simulink model "assignment4"  (R2017a)
settings: Solver=VariableStepAuto  StartTime=0.0  StopTime=10  RelTol=1e-3
undefined symbols (not defined in the file): sigbuilder_block
libraries: fl_lib x26, nesl_utility x24, pe_lib x11, elec_lib x6, powerlib_meascontrol x3
settings Model: Creator=hxx733  LastModifiedBy=super

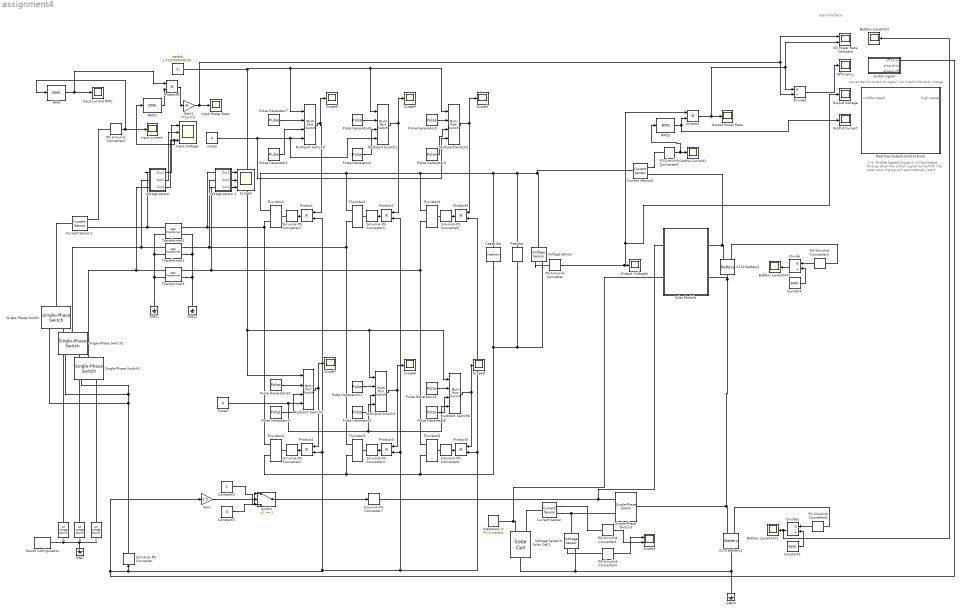
== system assignment4 ==
  note: User Interface
  note: remember to switch to signal 1 to check the solar charge
  note: high speed
  note: middle speed
  note: 1~2: Middle Speed Charge
      | 2~3:Fast Speed Charge
      | when the switch signal turned off,
      | the solar slow charge will automatically start.
  " Output Power Rate" : Scope
  " product " : Product
  2170 Battery1 : elec_lib/Sources/Battery  Vnom=3.7 V  R1=0.05 Ohm  prm_AH=2  AH=5.75 hr*A  V1=3 V  AH1=1.15 hr*A  prm_R2=1  R2=2000 Ohm  prm_fade=1  N_fade=100  AH_fade=45 hr*A  R1_fade=2.02 Ohm  V1_fade=10.35 V  i_specify=off  i_priority=None  i=0 A  i_nominal_specify=off  i_nominal_unit=A  i_nominal_value=1  v_specify=off  v_priority=None  v=0 V  v_nominal_specify=off  v_nominal_unit=V  v_nominal_value=1  charge_specify=on  charge_priority=High  charge=0 hr*A  charge_nominal_specify=off  charge_nominal_unit=hr*A  charge_nominal_value=1  num_cycles_specify=off  num_cycles_priority=High  num_cycles=0  num_cycles_nominal_specify=off  num_cycles_nominal_unit=1  num_cycles_nominal_value=1  thermal_mass=30000 J/K  Tmeas=298.15 K  Vnom_T2=12 V  R1_T2=2.2 Ohm  V1_T2=11.4 V  R2_T2=2200 Ohm  Tmeas2=273.15 K  temperature_specify=off  temperature_priority=High  temperature=298.15 K  temperature_nominal_specify=off  temperature_nominal_unit=K  temperature_nominal_value=1
      settings: SourceProductName=Simscape Electronics  SourceProductBaseCode=SN
  2170 Battery2 : elec_lib/Sources/Battery  Vnom=3.7 V  R1=0.05 Ohm  prm_AH=2  AH=5.75 hr*A  V1=3 V  AH1=1.15 hr*A  prm_R2=1  R2=2000 Ohm  prm_fade=1  N_fade=100  AH_fade=45 hr*A  R1_fade=2.02 Ohm  V1_fade=10.35 V  i_specify=off  i_priority=None  i=0 A  i_nominal_specify=off  i_nominal_unit=A  i_nominal_value=1  v_specify=off  v_priority=None  v=0 V  v_nominal_specify=off  v_nominal_unit=V  v_nominal_value=1  charge_specify=on  charge_priority=High  charge=0 hr*A  charge_nominal_specify=off  charge_nominal_unit=hr*A  charge_nominal_value=1  num_cycles_specify=off  num_cycles_priority=High  num_cycles=0  num_cycles_nominal_specify=off  num_cycles_nominal_unit=1  num_cycles_nominal_value=1  thermal_mass=30000 J/K  Tmeas=298.15 K  Vnom_T2=12 V  R1_T2=2.2 Ohm  V1_T2=11.4 V  R2_T2=2200 Ohm  Tmeas2=273.15 K  temperature_specify=off  temperature_priority=High  temperature=298.15 K  temperature_nominal_specify=off  temperature_nominal_unit=K  temperature_nominal_value=1
      settings: SourceProductName=Simscape Electronics  SourceProductBaseCode=SN
  A : fl_lib/Electrical/Electrical Sources/AC Voltage Source  amp=380/sqrt(3) V  shift=0 deg  frequency=50 Hz  omega=0 rad/s
  B : fl_lib/Electrical/Electrical Sources/AC Voltage Source  amp=380/sqrt(3) V  shift=120 deg  frequency=50 Hz  omega=0 rad/s
  Battery Level(Ah) : Scope
  Battery Level(Ah)1 : Scope
  Battery Level3(Ah) : Scope
  C : fl_lib/Electrical/Electrical Sources/AC Voltage Source  amp=380/sqrt(3) V  shift=240 deg  frequency=50 Hz  omega=0 rad/s
  Capacitor : elec_lib/Passive Devices/Capacitor  enable_table=0  c=100e-6 F  Cvec=[1.0e-5, 1.0e-6] F  Vvec=[0.0, 10.0] V  CV_table_symmetry=1  C_tol=5  enable_C_tol=0  tol_distribution=1  nSigma=4  r=1e-6 Ohm  g=0 1/Ohm  enable_operating_limits=0  operating_limit_action=2  max_working_voltage_range=[-25.0, 25.0] V  power_rating=1 W  enable_faults=0  fault_action=1  Cscale_faulted=100  R_faulted=1e-3 Ohm  G_faulted=0 1/Ohm  tau_fault=1e-3 s  enable_temporal_fault=0  t_fault=1 s  enable_behavioral_fault=0  max_permissible_voltage_range=[-100.0, 100.0] V  t_fail_on_voltage=1 s  i_specify=off  i_priority=None  i=0 A  i_nominal_specify=off  i_nominal_unit=A  i_nominal_value=1  v_specify=off  v_priority=None  v=0 V  v_nominal_specify=off  v_nominal_unit=V  v_nominal_value=1  vc_specify=off  vc_priority=High  vc=0 V  vc_nominal_specify=off  vc_nominal_unit=V  vc_nominal_value=1
  Constant : Constant  Value=3600
  Constant1 : Constant  Value=3600
  Constant2 : Constant
  Constant3 : Constant  Value=0
  Current Sensor : fl_lib/Electrical/Electrical Sensors/Current Sensor
  Current Sensor1 : fl_lib/Electrical/Electrical Sensors/Current Sensor
  Current Sensor2 : fl_lib/Electrical/Electrical Sensors/Current Sensor
  Divide : Product  Inputs=*/
  Divide1 : Product  Inputs=*/
  Divide2 : Product  Inputs=*/
  Efficiency : Scope
  GND{,1..2,4} (4 alike) : fl_lib/Electrical/Electrical Elements/Electrical Reference
  Gain : Gain  Gain=1.5
  Gain1 : Gain  Gain=3*sqrt(3)
  I/O Power Rate Compare : Scope  NumInputPorts=2
  Input Power Rate : Scope
  Input Voltage : Scope  NumInputPorts=3
  Input current : Scope
  Input current RMS : Scope
  "Irradiance, Ir" : fl_lib/Physical Signals/Sources/PS Constant  constant=1900*10
      settings: SourceProductName=Foundation Library
  Multiport Switch{1..6} (6 alike) : MultiPortSwitch
  OutPut Current : Scope
  OutPut Current1 : Scope
  Output Voltage : Scope
  Output Voltage1 : Scope
  PS-Simulink Converter{,1,3..4,6} (5 alike) : nesl_utility/PS-Simulink Converter  PhysicalDomain=network_engine_domain  SubClassName=ps_output  LeftPortType=input  RightPortType=output  PseudoPeriodic=off  Frequencies=[]  Unit=1  AffineConversion=off
  PS-Simulink Converter2 : nesl_utility/PS-Simulink Converter  PhysicalDomain=network_engine_domain  SubClassName=ps_output  LeftPortType=input  RightPortType=output  PseudoPeriodic=off  Frequencies=[]  Unit=C  AffineConversion=off
  PS-Simulink Converter5 : nesl_utility/PS-Simulink Converter  PhysicalDomain=network_engine_domain  SubClassName=ps_output  LeftPortType=input  RightPortType=output  PseudoPeriodic=off  Frequencies=[]  Unit=C  AffineConversion=off
  Product{,1..6} (7 alike) : Product
  Pulse Generator1 : DiscretePulseGenerator  PulseType=Time based  Period=1/50  PulseWidth=50
  Pulse Generator10 : DiscretePulseGenerator  PulseType=Time based  Period=1/50  PulseWidth=50  PhaseDelay=3/50/6++1/50/4
  Pulse Generator11 : DiscretePulseGenerator  PulseType=Time based  Period=1/50  PulseWidth=50  PhaseDelay=1/50/6+1/50/4
  Pulse Generator12 : DiscretePulseGenerator  PulseType=Time based  Period=1/50  PulseWidth=50  PhaseDelay=5/50/6+1/50/4
  Pulse Generator2 : DiscretePulseGenerator  PulseType=Time based  Period=1/50  PulseWidth=50  PhaseDelay=4/50/6
  Pulse Generator3 : DiscretePulseGenerator  PulseType=Time based  Period=1/50  PulseWidth=50  PhaseDelay=2/50/6
  Pulse Generator4 : DiscretePulseGenerator  PulseType=Time based  Period=1/50  PulseWidth=50  PhaseDelay=3/50/6
  Pulse Generator5 : DiscretePulseGenerator  PulseType=Time based  Period=1/50  PulseWidth=50  PhaseDelay=1/50/6
  Pulse Generator6 : DiscretePulseGenerator  PulseType=Time based  Period=1/50  PulseWidth=50  PhaseDelay=5/50/6
  Pulse Generator7 : DiscretePulseGenerator  PulseType=Time based  Period=1/50  PulseWidth=50  PhaseDelay=0+1/50/4
  Pulse Generator8 : DiscretePulseGenerator  PulseType=Time based  Period=1/50  PulseWidth=50  PhaseDelay=4/50/6+1/50/4
  Pulse Generator9 : DiscretePulseGenerator  PulseType=Time based  Period=1/50  PulseWidth=50  PhaseDelay=2/50/6+1/50/4
  RMS : powerlib_meascontrol/Measurements/RMS  TrueRMS=on  Freq=50  RMSInit=120  Ts=0
  RMS1 : powerlib_meascontrol/Measurements/RMS  TrueRMS=on  Freq=50  RMSInit=120  Ts=0
  RMS2 : powerlib_meascontrol/Measurements/RMS  TrueRMS=on  Freq=50  RMSInit=120  Ts=0
  Rectifier Output Control Knob : Subsystem  DialogController=hmiCreateDDGDialog  IsWebBlock=on  mask(MWDashboardBlock){webBlockId=5efd5572-5288-454e-8a17-a3fe679787e4, webBlockType=continuousknob, ShowInLibBrowser=on, ShowInitialText=on, HMISrcModelName=individualfinished}
      mask prompts: webBlockId "WebBlock Id"; webBlockType "WebBlock Type"; HMISrcModelName "Source Model"
      mask Help: helpview([docroot '/mapfiles/simulink.map'], 'hmi_knob')
      mask Display:
      | if strcmp(get_param(bdroot(gcb),'BlockDiagramType'), 'library')
      |     image([(matlabroot) '/toolbox/simulink/hmi/icons/ContinuousKnob.png']);
      | end
  Resistor : elec_lib/Passive Devices/Resistor  R=100 kOhm  R_tol=5  enable_R_tol=0  tol_distribution=1  nSigma=4  enable_operating_limits=0  operating_limit_action=2  max_working_voltage=100 V  power_rating=1 W  enable_faults=0  fault_action=1  R_faulted=inf Ohm  enable_temporal_fault=0  t_fault=1 s  enable_behavioral_fault=0  max_permissible_current=1 A  t_fail_on_current=1 s  noise_mode=0  sample_time=1e-3 s  repeatability=1  auto_seed=2769242599  user_seed=0  Tdevice=25 degC  alpha=3.93e-3 1/K  Tmeas=25 degC  thermal_mass=100 J/K  power_derating_T1=70 degC  power_derating_T2=155 degC  operating_temperature_range_vec=[-50.0, 150.0] degC  temperature_specify=off  temperature_priority=High  temperature=298.15 K  temperature_nominal_specify=off  temperature_nominal_unit=K  temperature_nominal_value=1
  Scope2 : Scope  NumInputPorts=3
  Scope3 : Scope  NumInputPorts=2
  Scope{4..9} (6 alike) : Scope
  Simulink-PS Converter{,1..7} (8 alike) : nesl_utility/Simulink-PS Converter  PhysicalDomain=network_engine_domain  SubClassName=ps_input  LeftPortType=input  RightPortType=output  PseudoPeriodic=off  Frequencies=[]  NoiseDistribution=none  NoiseParameters=[]  Unit=1  AffineConversion=off  FilteringAndDerivatives=provide  SimscapeFilterOrder=1  InputFilterTimeConstant=0.001  UdotUserProvided=0
  Single-Phase Switch{,1..3} (4 alike) : pe_lib/Switches & Breakers/Fundamental Components/Single-Phase Switch  R_closed=0.001 Ohm  G_open=1e-6 1/Ohm  threshold=0 V
      settings: SourceProductName=Simscape Power Systems  SourceProductBaseCode=PS
  Solar Cell1 : elec_lib/Sources/Solar Cell  prm=3  Isc=3.8 A  Voc=0.586 V  Is=3.15e-07 A  Is2=0 A  Iph=3.80 A  Ir0=1000 W/m^2  ec=1.4  N2=2  Rs=0.0042 Ohm  Rp=10.1 Ohm  N_series=700  TIPH1=0.000805 1/K  EG=1.14 eV  TXIS1=3.38  TXIS2=3  TRS1=0  TRP1=0  Tmeas=25 degC  TFIXED=30 degC  thermal_mass=100 J/K  initial_temperature=25 degC
      settings: SourceProductName=Simscape Electronics  SourceProductBaseCode=SN
  Solar Module : Subsystem
  Solver Configuration : nesl_utility/Solver Configuration  PhysicalDomain=network_engine_domain  SubClassName=solver  LeftPortType=input  RightPortType=generic  Accelerate=off  Tones=[]  Harmonics=[]  SimulateNoise=off  Profile=off  UseLocalSampling=off  EnableSwitchedLinearOptims=on  FrequencyDomain=off  UseCCode=off  RelTol=0.001  AbsTol=1e-06  MinStep=1e-09  ToWorkspace=off  RevertToSquareIcSolve=off  NumHomotopyIterations=100  PhasorMode=off  PhasorModeNumHarmonics=1  OverrideAbsTol=off  DoDC=off  ResidualTolerance=1e-09  UseLocalSolver=off  LocalSolverChoice=NE_BACKWARD_EULER_ADVANCER  LocalSolverSampleTime=0.001  DoFixedCost=off  MaxNonlinIter=3  MaxModeIter=2  LinearAlgebra=Sparse  DelaysMemoryBudget=1024  AutomaticFiltering=on  FilteringTimeConstant=0.001
  Switch : Switch  Threshold=1
  Thyristor{1..6} (6 alike) : pe_lib/Semiconductors/Fundamental Components/Thyristor  Vf=0.8 V  Ron=0.001 Ohm  Goff=1e-5 1/Ohm  Vgt=0.5 V  Ih=1 A  diode_param=1  diode_Vf=0.8 V  diode_Ron=0.001 Ohm  diode_Goff=1e-5 1/Ohm  diode_C=5e-8 F  diode_iRM=-235 A  diode_iF=300 A  diode_idot=-50 A/us  diode_trr_param=1  diode_trr_factor=3  diode_trr=15 us  diode_Qrr=1.5e+3 s*uA  thermal_loss_option=2  Voff=300 V  Tau=1e-4 s  Tj=[ 298.15 398.15 ] K  Iout_scalar=600 A  Eon_scalar=0.02286 J  Eoff_scalar=0.01714 J  Von_scalar=2.7 V  Iout_data=[ 0 10 50 100 200 400 600 ] A  Eon_data=[ 0 2.9e-4 0.00143 0.00286 0.00571 0.01314 0.02286; 0 5.7e-4 0.00263 0.00514 0.01029 0.02057 0.03029 ] J  Eoff_data=[ 0 2.1e-4 0.00107 0.00214 0.00429 0.009859999999999999 0.01714; 0 4.3e-4 0.00197 0.00386 0.00771 0.01543 0.02271 ] J  Von_data=[ 0 1.1 1.3 1.45 1.75 2.25 2.7; 0 1 1.15 1.35 1.7 2.35 3 ] V
      settings: SourceProductName=Simscape Power Systems  SourceProductBaseCode=PS
  Transformer1 : fl_lib/Electrical/Electrical Elements/Ideal Transformer  n=1:1  i1_specify=off  i1_priority=None  i1=0 A  i1_nominal_specify=off  i1_nominal_unit=A  i1_nominal_value=1  v1_specify=off  v1_priority=None  v1=0 V  v1_nominal_specify=off  v1_nominal_unit=V  v1_nominal_value=1  i2_specify=off  i2_priority=None  i2=0 A  i2_nominal_specify=off  i2_nominal_unit=A  i2_nominal_value=1  v2_specify=off  v2_priority=None  v2=0 V  v2_nominal_specify=off  v2_nominal_unit=V  v2_nominal_value=1
      settings: SourceProductName=Simscape  SourceProductBaseCode=SS
  Transformer2 : fl_lib/Electrical/Electrical Elements/Ideal Transformer  n=1:1  i1_specify=off  i1_priority=None  i1=0 A  i1_nominal_specify=off  i1_nominal_unit=A  i1_nominal_value=1  v1_specify=off  v1_priority=None  v1=0 V  v1_nominal_specify=off  v1_nominal_unit=V  v1_nominal_value=1  i2_specify=off  i2_priority=None  i2=0 A  i2_nominal_specify=off  i2_nominal_unit=A  i2_nominal_value=1  v2_specify=off  v2_priority=None  v2=0 V  v2_nominal_specify=off  v2_nominal_unit=V  v2_nominal_value=1
      settings: SourceProductName=Simscape  SourceProductBaseCode=SS
  Transformer3 : fl_lib/Electrical/Electrical Elements/Ideal Transformer  n=1:1  i1_specify=off  i1_priority=None  i1=0 A  i1_nominal_specify=off  i1_nominal_unit=A  i1_nominal_value=1  v1_specify=off  v1_priority=None  v1=0 V  v1_nominal_specify=off  v1_nominal_unit=V  v1_nominal_value=1  i2_specify=off  i2_priority=None  i2=0 A  i2_nominal_specify=off  i2_nominal_unit=A  i2_nominal_value=1  v2_specify=off  v2_priority=None  v2=0 V  v2_nominal_specify=off  v2_nominal_unit=V  v2_nominal_value=1
      settings: SourceProductName=Simscape  SourceProductBaseCode=SS
  Voltage Sensor : fl_lib/Electrical/Electrical Sensors/Voltage Sensor
  Voltage Sensor4 : fl_lib/Electrical/Electrical Sensors/Voltage Sensor
  none1 : Constant  Value=0
  none2 : Constant  Value=0
  switch : Constant  Value=2.4320085608106
  switch signal : Subsystem  Tag=STV Subsys  LoadFcn=sigbuilder_block('load');  StartFcn=sigbuilder_block('start');  StopFcn=sigbuilder_block('stop');  ClipboardFcn=sigbuilder_block('clipboard');  mask(Sigbuilder block){tuvar=[0:10]}
      mask help: Simulink:masks:SigbuilderBlock_MD
      mask init:
      | if ~strcmp(get_param(bdroot(gcbh),'SimulationStatus'),'stopped') tuvar = sigbuilder_block('maskInit'); end
      settings: CopyFcn=sigbuilder_block('copy');  DeleteFcn=sigbuilder_block('delete');  ModelCloseFcn=sigbuilder_block('modelClose');  PreSaveFcn=sigbuilder_block('preSave');  PauseFcn=sigbuilder_block('pause');  ContinueFcn=sigbuilder_block('continue');  NameChangeFcn=sigbuilder_block('namechange');  OpenFcn=sigbuilder_block('open',[442.125 105 550.5 400.125 ]);  CloseFcn=sigbuilder_block('close');
      mask Display: plot(0, 0, 100, 100,[2, 2, 32, 32, 2], [68, 8, 8, 68, 68],[32, 2], [38, 38], [32, 19, 2],[53, 60, 44], [32, 17, 17, 2],[16, 16, 31, 31]);txt = getActiveGroup(gcbh);text(2, 100, txt,'verticalAlignment', 'top');
  "voltage sensor " : Subsystem
  voltage sensor 1 : Subsystem
  wires:
  PS-Simulink Converter/1 -> Output Voltage/1, " product "/1, Output Voltage1/1
  PS-Simulink Converter4/1 -> Scope3/1
  "voltage sensor "/1(Out1) -> Input Voltage/1
  "voltage sensor "/2(Out2) -> Input Voltage/2
  "voltage sensor "/3(Out3) -> RMS1/1, Input Voltage/3
  PS-Simulink Converter1/1 -> Scope3/2
  Product/1 -> Simulink-PS Converter1/1
  Product1/1 -> Simulink-PS Converter2/1
  Product2/1 -> Simulink-PS Converter3/1
  Product3/1 -> Simulink-PS Converter4/1
  Product4/1 -> Simulink-PS Converter5/1
  Product5/1 -> Simulink-PS Converter6/1
  Divide/1 -> Battery Level3(Ah)/1
  PS-Simulink Converter5/1 -> Divide/1
  Constant/1 -> Divide/2
  PS-Simulink Converter2/1 -> Divide1/1
  Constant1/1 -> Divide1/2
  Divide1/1 -> Battery Level(Ah)/1, Battery Level(Ah)1/1
  Multiport Switch1/1 -> Product2/1, Scope4/1
  Pulse Generator2/1 -> Multiport Switch1/3
  Pulse Generator8/1 -> Multiport Switch1/2
  Pulse Generator3/1 -> Multiport Switch2/3
  Pulse Generator9/1 -> Multiport Switch2/2
  Multiport Switch2/1 -> Product4/1, Scope5/1
  none1/1 -> Multiport Switch2/4, Multiport Switch1/4, Multiport Switch3/4
  Multiport Switch3/1 -> Product/1, Scope6/1
  Pulse Generator1/1 -> Multiport Switch3/3
  Pulse Generator7/1 -> Multiport Switch3/2
  Multiport Switch4/1 -> Product1/1, Scope7/1
  none2/1 -> Multiport Switch4/4, Multiport Switch6/4, Multiport Switch5/4
  Pulse Generator10/1 -> Multiport Switch4/2
  Pulse Generator4/1 -> Multiport Switch4/3
  Multiport Switch5/1 -> Product3/1, Scope8/1
  Pulse Generator11/1 -> Multiport Switch5/2
  Pulse Generator5/1 -> Multiport Switch5/3
  Multiport Switch6/1 -> Product5/1, Scope9/1
  Pulse Generator12/1 -> Multiport Switch6/2
  Pulse Generator6/1 -> Multiport Switch6/3
  voltage sensor 1/1(Out1) -> Scope2/1
  voltage sensor 1/3(Out3) -> Scope2/3
  voltage sensor 1/2(Out2) -> Scope2/2
  Constant3/1 -> Switch/1
  Constant2/1 -> Switch/3
  Gain/1 -> Switch/2
  switch signal/1(off to on) -> Gain/1, Product/2, Product1/2, Product2/2, Product3/2, Product4/2, Product5/2, Simulink-PS Converter/1
  switch/1 -> Multiport Switch4/1, Multiport Switch6/1, Multiport Switch5/1, Multiport Switch3/1, Multiport Switch2/1, Multiport Switch1/1
  Switch/1 -> Simulink-PS Converter7/1
  PS-Simulink Converter3/1 -> RMS/1, Input current/1
  Product6/1 -> Gain1/1
  Gain1/1 -> Divide2/2, I/O Power Rate Compare/1, Input Power Rate/1
  PS-Simulink Converter6/1 -> RMS2/1, OutPut Current1/1
  " product "/1 -> Divide2/1, I/O Power Rate Compare/2, " Output Power Rate"/1
  Divide2/1 -> Efficiency/1
  RMS/1 -> Product6/1, Input current RMS/1
  RMS1/1 -> Product6/2
  RMS2/1 -> " product "/2, OutPut Current/1
  connections:
  B/RConn1 -- Solver Configuration/RConn1 -- A/RConn1 -- C/RConn1 -- GND/LConn1
  GND1/LConn1 -- Transformer3/LConn2 -- Transformer1/LConn2 -- Transformer2/LConn2
  Transformer2/RConn2 -- Transformer1/RConn2 -- Transformer3/RConn2 -- GND2/LConn1
  "voltage sensor "/LConn2 -- Single-Phase Switch1/RConn1 -- Transformer2/LConn1
  "voltage sensor "/LConn1 -- Transformer1/LConn1 -- Current Sensor1/RConn2
  Thyristor1/RConn1 -- voltage sensor 1/LConn1 -- Transformer1/RConn1 -- Thyristor4/RConn2
  Thyristor2/RConn1 -- voltage sensor 1/LConn2 -- Transformer2/RConn1 -- Thyristor5/RConn2
  Thyristor3/RConn1 -- Transformer3/RConn1 -- voltage sensor 1/LConn3 -- Thyristor6/RConn2
  Thyristor4/RConn1 -- Thyristor5/RConn1 -- Voltage Sensor/RConn2 -- Resistor/RConn1 -- Capacitor/RConn1 -- Thyristor6/RConn1
  Voltage Sensor/RConn1 -- PS-Simulink Converter/LConn1
  Solar Module/LConn2 -- Solar Cell1/LConn1 -- "Irradiance, Ir"/RConn1
  Voltage Sensor4/RConn1 -- PS-Simulink Converter4/LConn1
  Voltage Sensor/LConn1 -- Current Sensor2/LConn1 -- Resistor/LConn1 -- Thyristor1/RConn2 -- Thyristor2/RConn2 -- Thyristor3/RConn2 -- Capacitor/LConn1
  Voltage Sensor4/RConn2 -- Solar Cell1/RConn1 -- 2170 Battery2/RConn1 -- GND4/LConn1
  2170 Battery2/LConn1 -- Solar Module/RConn2 -- 2170 Battery1/RConn1 -- Single-Phase Switch3/RConn1
  "voltage sensor "/LConn3 -- Single-Phase Switch2/RConn1 -- Transformer3/LConn1
  Current Sensor/LConn1 -- Solar Cell1/LConn2
  Current Sensor/RConn1 -- PS-Simulink Converter1/LConn1
  A/LConn1 -- Single-Phase Switch/LConn2
  B/LConn1 -- Single-Phase Switch1/LConn2
  Single-Phase Switch2/LConn2 -- C/LConn1
  Simulink-PS Converter/RConn1 -- Single-Phase Switch2/LConn1 -- Single-Phase Switch1/LConn1 -- Single-Phase Switch/LConn1
  Simulink-PS Converter1/RConn1 -- Thyristor1/LConn1
  Simulink-PS Converter2/RConn1 -- Thyristor4/LConn1
  Simulink-PS Converter3/RConn1 -- Thyristor2/LConn1
  Simulink-PS Converter4/RConn1 -- Thyristor5/LConn1
  Simulink-PS Converter5/RConn1 -- Thyristor3/LConn1
  Simulink-PS Converter6/RConn1 -- Thyristor6/LConn1
  2170 Battery1/LConn2 -- PS-Simulink Converter5/LConn1
  Current Sensor/RConn2 -- Single-Phase Switch3/LConn2 -- Voltage Sensor4/LConn1
  2170 Battery2/LConn2 -- PS-Simulink Converter2/LConn1
  Simulink-PS Converter7/RConn1 -- Solar Module/LConn1 -- Single-Phase Switch3/LConn1
  Current Sensor1/LConn1 -- Single-Phase Switch/RConn1
  Current Sensor1/RConn1 -- PS-Simulink Converter3/LConn1
  Solar Module/RConn1 -- Current Sensor2/RConn2 -- 2170 Battery1/LConn1
  Current Sensor2/RConn1 -- PS-Simulink Converter6/LConn1

== system assignment4/Rectifier Output Control Knob ==

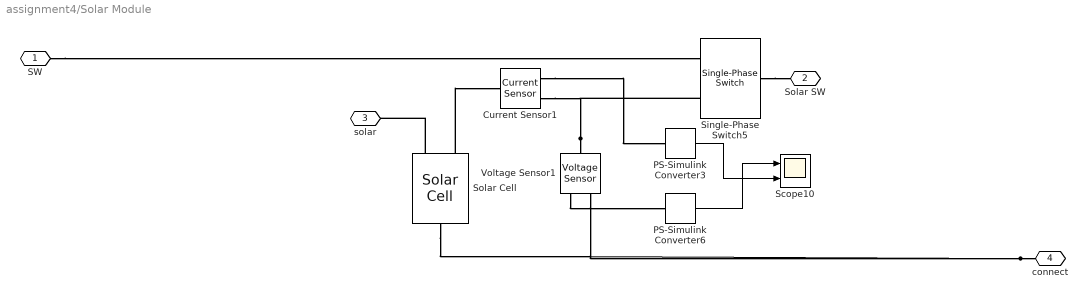
== system assignment4/Solar Module ==
  Current Sensor1 : fl_lib/Electrical/Electrical Sensors/Current Sensor
  PS-Simulink Converter3 : nesl_utility/PS-Simulink Converter  PhysicalDomain=network_engine_domain  SubClassName=ps_output  LeftPortType=input  RightPortType=output  PseudoPeriodic=off  Frequencies=[]  Unit=1  AffineConversion=off
  PS-Simulink Converter6 : nesl_utility/PS-Simulink Converter  PhysicalDomain=network_engine_domain  SubClassName=ps_output  LeftPortType=input  RightPortType=output  PseudoPeriodic=off  Frequencies=[]  Unit=1  AffineConversion=off
  Scope10 : Scope  NumInputPorts=2
  Single-Phase Switch5 : pe_lib/Switches & Breakers/Fundamental Components/Single-Phase Switch  R_closed=0.001 Ohm  G_open=1e-6 1/Ohm  threshold=0 V
      settings: SourceProductName=Simscape Power Systems  SourceProductBaseCode=PS
  Solar Cell : elec_lib/Sources/Solar Cell  prm=3  Isc=3.8 A  Voc=0.586 V  Is=3.15e-07 A  Is2=0 A  Iph=3.80 A  Ir0=1000 W/m^2  ec=1.4  N2=2  Rs=0.0042 Ohm  Rp=10.1 Ohm  N_series=700  TIPH1=0.000805 1/K  EG=1.14 eV  TXIS1=3.38  TXIS2=3  TRS1=0  TRP1=0  Tmeas=25 degC  TFIXED=30 degC  thermal_mass=100 J/K  initial_temperature=25 degC
      settings: SourceProductName=Simscape Electronics  SourceProductBaseCode=SN
  Voltage Sensor1 : fl_lib/Electrical/Electrical Sensors/Voltage Sensor
  SW : PMIOPort  Port=1  Side=Left
  Solar SW : PMIOPort  Port=2  Side=Right
  solar : PMIOPort  Port=3  Side=Left
  connect : PMIOPort  Port=4  Side=Right
  wires:
  PS-Simulink Converter3/1 -> Scope10/2
  PS-Simulink Converter6/1 -> Scope10/1
  connections:
  Voltage Sensor1/RConn1 -- PS-Simulink Converter6/LConn1
  Voltage Sensor1/LConn1 -- Current Sensor1/RConn2 -- Single-Phase Switch5/LConn2
  Solar Cell/LConn2 -- Current Sensor1/LConn1
  SW/RConn1 -- Single-Phase Switch5/LConn1
  Current Sensor1/RConn1 -- PS-Simulink Converter3/LConn1
  connect/RConn1 -- Solar Cell/RConn1 -- Voltage Sensor1/RConn2
  Solar Cell/LConn1 -- solar/RConn1
  Single-Phase Switch5/RConn1 -- Solar SW/RConn1

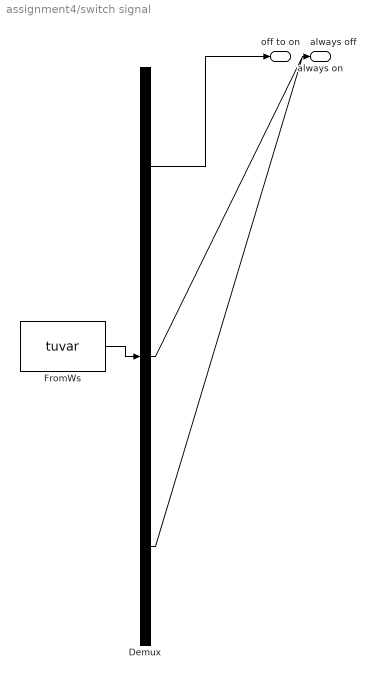
== system assignment4/switch signal ==
  Demux : Demux  Tag=STV Demux  Outputs=3
  FromWs : FromWorkspace  Tag=STV FromWs  VariableName=tuvar  SampleTime=0
      SigBuilderData=|
      | common.afterFinalStr = 'Extrapolate'
      | common.sampleTime = 0
      | dataSet.timeRange = [0 10]
      | dataSet.name = 'Group 1'
      | sbobj.Groups.Name = 'Group 1'
      | sbobj.Groups.Signals(1).Name = 'off to on'
      | sbobj.Groups.Signals(1).XData = [0 5 5 6 10]
      | sbobj.Groups.Signals(1).YData = [0 0 0.995 0.995 0.995]
      | sbobj.Groups.Signals(2).Name = 'always on'
      | sbobj.Groups.Signals(2).XData = [0 10]
      | sbobj.Groups.Signals(2).YData = [1 1]
      | sbobj.Groups.Signals(3).Name = 'always off'
      | sbobj.Groups.Signals(3).XData = [0 10]
      | sbobj.Groups.Signals(3).YData = [0 0]
  off to on : Outport  Tag=STV Outport
  always on : Outport  Tag=STV Outport  Port=2
  always off : Outport  Tag=STV Outport  Port=3
  wires:
  Demux/1 -> off to on/1
  FromWs/1 -> Demux/1
  Demux/2 -> always on/1
  Demux/3 -> always off/1

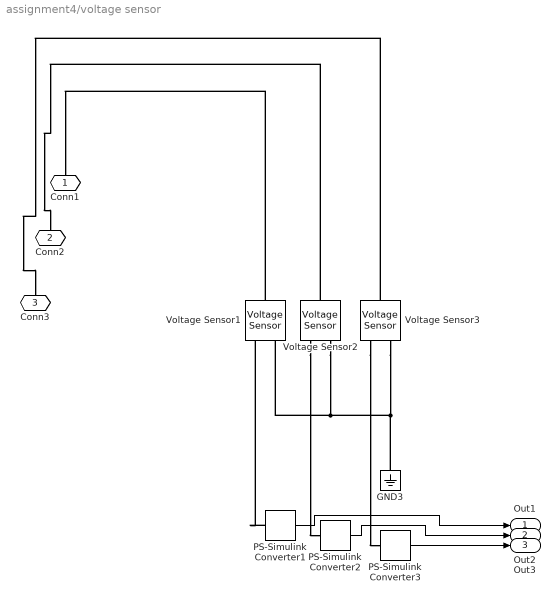
== system assignment4/voltage sensor  ==
  GND3 : fl_lib/Electrical/Electrical Elements/Electrical Reference
  PS-Simulink Converter1 : nesl_utility/PS-Simulink Converter  PhysicalDomain=network_engine_domain  SubClassName=ps_output  LeftPortType=input  RightPortType=output  PseudoPeriodic=off  Frequencies=[]  Unit=1  AffineConversion=off
  PS-Simulink Converter2 : nesl_utility/PS-Simulink Converter  PhysicalDomain=network_engine_domain  SubClassName=ps_output  LeftPortType=input  RightPortType=output  PseudoPeriodic=off  Frequencies=[]  Unit=1  AffineConversion=off
  PS-Simulink Converter3 : nesl_utility/PS-Simulink Converter  PhysicalDomain=network_engine_domain  SubClassName=ps_output  LeftPortType=input  RightPortType=output  PseudoPeriodic=off  Frequencies=[]  Unit=1  AffineConversion=off
  Voltage Sensor1 : fl_lib/Electrical/Electrical Sensors/Voltage Sensor
  Voltage Sensor2 : fl_lib/Electrical/Electrical Sensors/Voltage Sensor
  Voltage Sensor3 : fl_lib/Electrical/Electrical Sensors/Voltage Sensor
  Conn1 : PMIOPort  Port=1  Side=Left
  Conn2 : PMIOPort  Port=2  Side=Left
  Conn3 : PMIOPort  Port=3  Side=Left
  Out1 : Outport
  Out2 : Outport  Port=2
  Out3 : Outport  Port=3
  wires:
  PS-Simulink Converter1/1 -> Out1/1
  PS-Simulink Converter2/1 -> Out2/1
  PS-Simulink Converter3/1 -> Out3/1
  connections:
  Voltage Sensor3/LConn1 -- Conn3/RConn1
  GND3/LConn1 -- Voltage Sensor2/RConn2 -- Voltage Sensor1/RConn2 -- Voltage Sensor3/RConn2
  PS-Simulink Converter1/LConn1 -- Voltage Sensor1/RConn1
  Voltage Sensor2/RConn1 -- PS-Simulink Converter2/LConn1
  Voltage Sensor3/RConn1 -- PS-Simulink Converter3/LConn1
  Voltage Sensor2/LConn1 -- Conn2/RConn1
  Voltage Sensor1/LConn1 -- Conn1/RConn1

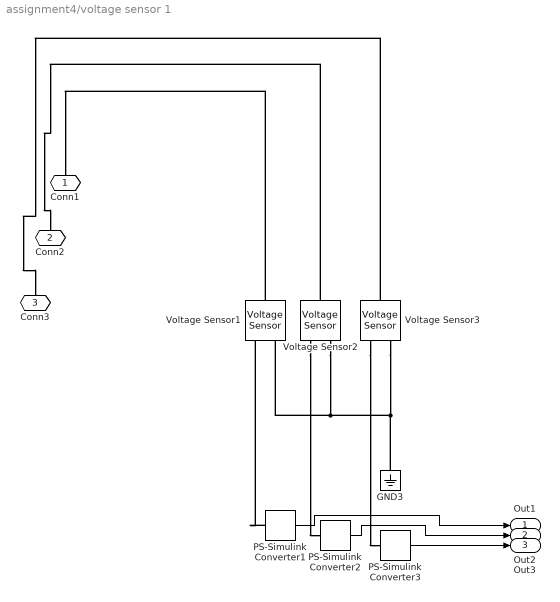
== system assignment4/voltage sensor 1 ==
  GND3 : fl_lib/Electrical/Electrical Elements/Electrical Reference
  PS-Simulink Converter1 : nesl_utility/PS-Simulink Converter  PhysicalDomain=network_engine_domain  SubClassName=ps_output  LeftPortType=input  RightPortType=output  PseudoPeriodic=off  Frequencies=[]  Unit=1  AffineConversion=off
  PS-Simulink Converter2 : nesl_utility/PS-Simulink Converter  PhysicalDomain=network_engine_domain  SubClassName=ps_output  LeftPortType=input  RightPortType=output  PseudoPeriodic=off  Frequencies=[]  Unit=1  AffineConversion=off
  PS-Simulink Converter3 : nesl_utility/PS-Simulink Converter  PhysicalDomain=network_engine_domain  SubClassName=ps_output  LeftPortType=input  RightPortType=output  PseudoPeriodic=off  Frequencies=[]  Unit=1  AffineConversion=off
  Voltage Sensor1 : fl_lib/Electrical/Electrical Sensors/Voltage Sensor
  Voltage Sensor2 : fl_lib/Electrical/Electrical Sensors/Voltage Sensor
  Voltage Sensor3 : fl_lib/Electrical/Electrical Sensors/Voltage Sensor
  Conn1 : PMIOPort  Port=1  Side=Left
  Conn2 : PMIOPort  Port=2  Side=Left
  Conn3 : PMIOPort  Port=3  Side=Left
  Out1 : Outport
  Out2 : Outport  Port=2
  Out3 : Outport  Port=3
  wires:
  PS-Simulink Converter1/1 -> Out1/1
  PS-Simulink Converter2/1 -> Out2/1
  PS-Simulink Converter3/1 -> Out3/1
  connections:
  Voltage Sensor3/LConn1 -- Conn3/RConn1
  GND3/LConn1 -- Voltage Sensor2/RConn2 -- Voltage Sensor1/RConn2 -- Voltage Sensor3/RConn2
  PS-Simulink Converter1/LConn1 -- Voltage Sensor1/RConn1
  Voltage Sensor2/RConn1 -- PS-Simulink Converter2/LConn1
  Voltage Sensor3/RConn1 -- PS-Simulink Converter3/LConn1
  Voltage Sensor2/LConn1 -- Conn2/RConn1
  Voltage Sensor1/LConn1 -- Conn1/RConn1
